simulink model "Problem_5"  (R2020b)
settings: Solver=VariableStepAuto  StartTime=0.0  StopTime=10  RelTol=1e-3
settings Model: Creator=HP  LastModifiedBy=HP

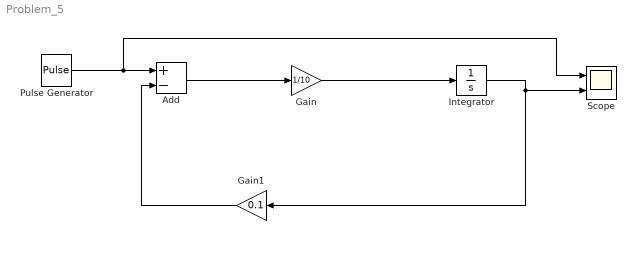
== system Problem_5 ==
  Add : Sum  Inputs=+-
  Gain : Gain  Gain=1/10
  Gain1 : Gain  Gain=0.1
  Integrator : Integrator
  Pulse Generator : DiscretePulseGenerator  PulseType=Time based  Period=1  PulseWidth=5
  Scope : Scope  NumInputPorts=2
  wires:
  Gain1/1 -> Add/2
  Gain/1 -> Integrator/1
  Add/1 -> Gain/1
  Integrator/1 -> Gain1/1, Scope/2
  Pulse Generator/1 -> Scope/1, Add/1
